simulink model "buck_pv"  (R2024a)
settings: Solver=FixedStepDiscrete  StartTime=0  StopTime=0.3  FixedStep=(1/150000)/100  RelTol=1e-3
model workspace (MAT data in the model file):
  Var = 20
values from neighbouring files (symbols this model uses):
  ki_0 = -mk*sin(thetak)*wcg_f    [Projeto_PI_Buck_PV_200W.m]    (also in Projeto_PI_Buck_PV_330W.m)
  kp_0 = mk*cos(thetak)    [Projeto_PI_Buck_PV_200W.m]    (also in Projeto_PI_Buck_PV_330W.m)
libraries: spsSeriesRLCBranchLib x6, spsDiodeLib x4, spsMeanLib x4, spsCurrentMeasurementLib x2, spsDCVoltageSourceLib x2, spsGroundLib x2, spsMosfetLib x2, spsPVArrayLib x2, spsPWMGeneratorDCDCLib x2, spsVoltageMeasurementLib x2, fuzblock x1, spspowerguiLib x1
settings Model: Creator=mario  LastModifiedBy=mario
settings SolverCC: MaxConsecutiveMinStep=10  ZeroCrossAlgorithm=Adaptive  SolverResetMethod=Robust
settings DebuggingCC: IgnoredZcDiagnostic=none
settings ModelReferenceCC: EnableRefExpFcnMdlSchedulingChecks=on
settings RTWCC: GPUComputeCapability=3.5

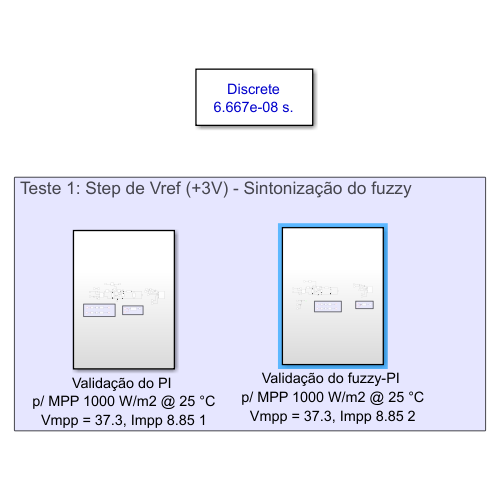
[thumbnail: Simulink's stored preview of the top-level diagram]
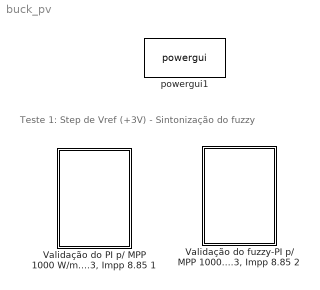
== system buck_pv ==
  note: Teste 1: Step de Vref (+3V) - Sintonização do fuzzy
  "Validação do PI p/ MPP 1000 W/m2 @ 25 °C Vmpp = 37.3, Impp 8.85 1" : Subsystem
  "Validação do fuzzy-PI p/ MPP 1000 W/m2 @ 25 °C Vmpp = 37.3, Impp 8.85 2" : Subsystem
  powergui1 : spspowerguiLib/powergui  Priority=1  SimulationMode=Discrete  SampleTime=(1/150000)/100  frequency=60  Iterations=50  frequencyindice=0  Pbase=100e6  ErrMax=1e-4  UnitsV=kV  UnitsW=MW  buscounter=0  FunctionMessages=off  echomessages=off  EnableUseOfTLC=off  CurrentSourceSwitches=off  DisableSnubberDevices=on  DisableRonSwitches=off  DisableVfSwitches=off  DisplayEquations=off  AutomaticDiscreteSolvers=off  SolverType=Tustin/Backward Euler (TBE)  Interpol=off  ExternalGateDelay=off  methode=off  Ts=100  x0status=blocks  SPID=on  SwTol=0  HookPort=off  NonlinearTolerance=1e-4  nMaxIteration=100  ContinueOnMaxIteration=on  RestoreLinks=warning  ResistiveCurrentMeasurement=off  Frange=[0:2:500]  Ylog=off  Xlog=on  ShowGrid=off  save=off  variable=ZData  structure=0  ZoomFFT=off  StartTime=0.0  cycles=1  DisplayStyle=1  fundamental=60  FreqAxis=off  MaxFrequency=1000  frequencyindicesteady=1  RmsSteady=1  display=off

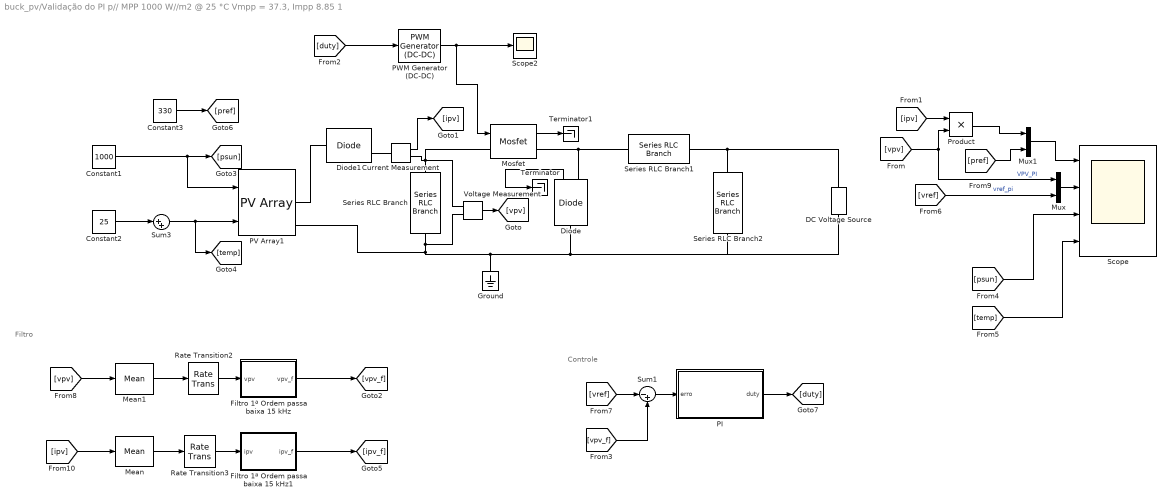
== system buck_pv/Validação do PI p// MPP 1000 W//m2 @ 25 °C Vmpp = 37.3, Impp 8.85 1 ==
  note: Controle
  note: Filtro
  Constant1 : Constant  Value=1000
  Constant2 : Constant  Value=25
  Constant3 : Constant  Value=330
  Current Measurement : spsCurrentMeasurementLib/Current Measurement  PhasorSimulation=off  OutputType=Complex  PSBequivalent=0
  DC Voltage Source : spsDCVoltageSourceLib/DC Voltage Source  Amplitude=12  Measurements=None
  Diode : spsDiodeLib/Diode  Ron=0.001  Lon=0  Vf=1  IC=0  UseSnubber=0  Rs=500  Cs=250e-9  Measurements=on
  Diode1 : spsDiodeLib/Diode  Ron=0.001  Lon=0  Vf=0.001  IC=0  UseSnubber=0  Rs=500  Cs=250e-9  Measurements=on
  Filtro 1ª Ordem passa baixa 15 kHz : MATLAB Function  TreatAsAtomicUnit=on
  Filtro 1ª Ordem passa baixa 15 kHz1 : MATLAB Function  TreatAsAtomicUnit=on
  Ground : spsGroundLib/Ground  LConnTagsString=a
  Mean : spsMeanLib/Mean  Freq=150e3  Vinit=0  Ts=(1/150000)/100
  Mean1 : spsMeanLib/Mean  Freq=150e3  Vinit=0  Ts=(1/150000)/100
  Mosfet : spsMosfetLib/Mosfet  Ron=6.5e-3  Lon=0  Rd=0.01  Vfd=0  IC=0  Rs=1e5  Cs=inf  Measurements=on
  Mux : Mux  Inputs=2
  Mux1 : Mux  Inputs=2
  PI : Subsystem
  PV Array1 : spsPVArrayLib/PV Array  Npar=1  Nser=1  PlotType=array @ 25 deg.C & specified irradiances  S_vec="[ 1000  800 600 400 200]"  Temp_C_vec=[ 50 40 30 20 10 ]  ModuleName=User-defined  PlotWhenSelected=off  Pm=330.105  Ncell=72  Voc=46.1  Isc=9.29  Vm=37.3  Im=8.85  beta_Voc_pc=-0.32  alpha_Isc_pc=0.05  beta_Voc=-0.14752  alpha_Isc=0.004645  IL=9.3231  I0=7.1464e-11  nI=0.97384  Rsh=1329.6875  Rs=0.38666  RobustModel=off  RobustCellTemperature=313.3991  BAL=on  Tc=1e-7  Tfilter=5e-5
  PWM Generator (DC-DC) : spsPWMGeneratorDCDCLib/PWM Generator (DC-DC)  Fsw=150000  Ts=1e-7
  Product : Product
  Rate Transition2 : RateTransition  OutPortSampleTime=1/150000
  Rate Transition3 : RateTransition  OutPortSampleTime=1/150000
  Scope : Scope  NumInputPorts=4
  Scope2 : Scope
  Series RLC Branch : spsSeriesRLCBranchLib/Series RLC Branch  LConnTagsString=__new0  RConnTagsString=__new0  BranchType=RC  Resistance=6.519e-3  Inductance=1e-3  SetiL0=off  InitialCurrent=0  Capacitance=2.7e-3  Setx0=off  InitialVoltage=37.3  Measurements=None
  Series RLC Branch1 : spsSeriesRLCBranchLib/Series RLC Branch  LConnTagsString=__new0  RConnTagsString=__new0  BranchType=RL  Resistance=3e-3  Inductance=22.109e-6  SetiL0=off  InitialCurrent=25.8056  Capacitance=1e-6  Setx0=off  InitialVoltage=0  Measurements=None
  Series RLC Branch2 : spsSeriesRLCBranchLib/Series RLC Branch  LConnTagsString=__new0  RConnTagsString=__new0  BranchType=RC  Resistance=35.2e-3  Inductance=1e-3  SetiL0=off  InitialCurrent=0  Capacitance=500e-6  Setx0=off  InitialVoltage=12  Measurements=None
  Sum1 : Sum  Inputs=|-+
  Sum3 : Sum  Inputs=|++
  Terminator : Terminator
  Terminator1 : Terminator
  Voltage Measurement : spsVoltageMeasurementLib/Voltage Measurement  PhasorSimulation=off  OutputType=Complex  PSBequivalent=0
  wires:
  Mux1/1 -> Scope/1
  [ipv] -> Product/1
  PWM Generator (DC-DC)/1 -> Scope2/1, Mosfet/1
  [vpv] -> Product/2, Mux/1  "VPV_PI"
  [duty] -> PWM Generator (DC-DC)/1
  Product/1 -> Mux1/1
  [pref] -> Mux1/2
  [psun] -> Scope/3
  [vref] -> Mux/2  "vref_pi"
  [temp] -> Scope/4
  Mux/1 -> Scope/2
  Diode/1 -> Terminator/1
  Mosfet/1 -> Terminator1/1
  Constant3/1 -> [pref]
  Voltage Measurement/1 -> [vpv]
  Current Measurement/1 -> [ipv]
  [vpv_f] -> Sum1/2
  [vref] -> Sum1/1
  Sum3/1 -> PV Array1/2, [temp]
  Constant2/1 -> Sum3/1
  Constant1/1 -> PV Array1/1, [psun]
  Sum1/1 -> PI/1(erro)
  PI/1(duty) -> [duty]
  Filtro 1ª Ordem passa baixa 15 kHz1/1(ipv_f) -> [ipv_f]
  Mean1/1 -> Rate Transition2/1
  Rate Transition2/1 -> Filtro 1ª Ordem passa baixa 15 kHz/1(vpv)
  Rate Transition3/1 -> Filtro 1ª Ordem passa baixa 15 kHz1/1(ipv)
  [vpv] -> Mean1/1
  Filtro 1ª Ordem passa baixa 15 kHz/1(vpv_f) -> [vpv_f]
  Mean/1 -> Rate Transition3/1
  [ipv] -> Mean/1
  connections:
  Series RLC Branch1/RConn1 -- DC Voltage Source/RConn1 -- Series RLC Branch2/LConn1
  Mosfet/LConn1 -- Current Measurement/RConn1 -- Voltage Measurement/LConn1 -- Series RLC Branch/LConn1
  DC Voltage Source/LConn1 -- Series RLC Branch2/RConn1 -- Diode/LConn1 -- Ground/LConn1 -- PV Array1/RConn2 -- Voltage Measurement/LConn2 -- Series RLC Branch/RConn1
  Mosfet/RConn1 -- Series RLC Branch1/LConn1 -- Diode/RConn1
  Diode1/RConn1 -- Current Measurement/LConn1
  PV Array1/RConn1 -- Diode1/LConn1

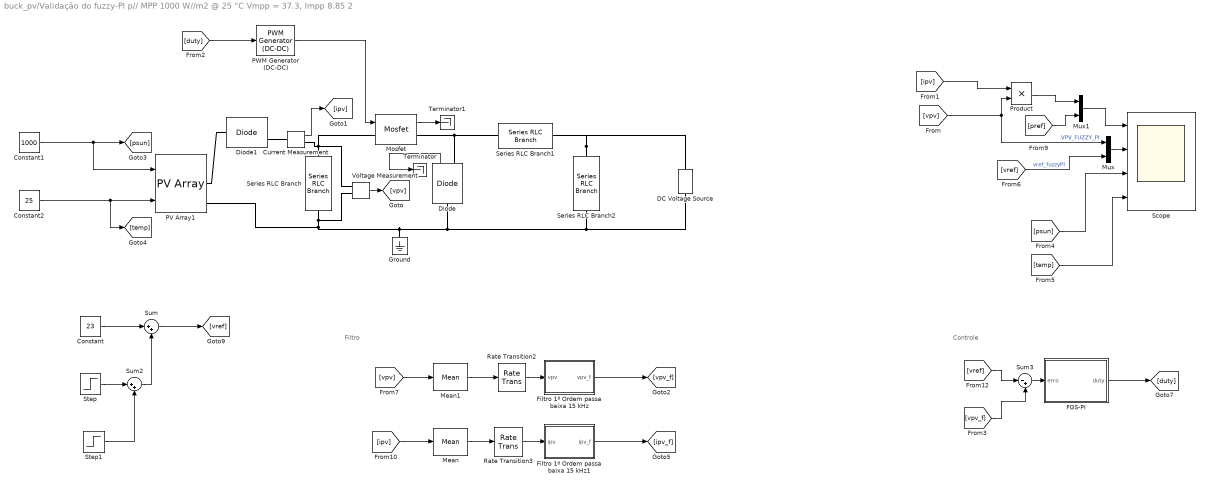
== system buck_pv/Validação do fuzzy-PI p// MPP 1000 W//m2 @ 25 °C Vmpp = 37.3, Impp 8.85 2 ==
  note: Controle
  note: Filtro
  Constant : Constant  Value=23
  Constant1 : Constant  Value=1000
  Constant2 : Constant  Value=25
  Current Measurement : spsCurrentMeasurementLib/Current Measurement  PhasorSimulation=off  OutputType=Complex  PSBequivalent=0
  DC Voltage Source : spsDCVoltageSourceLib/DC Voltage Source  Amplitude=12  Measurements=None
  Diode : spsDiodeLib/Diode  Ron=0.001  Lon=0  Vf=1  IC=0  UseSnubber=0  Rs=500  Cs=250e-9  Measurements=on
  Diode1 : spsDiodeLib/Diode  Ron=0.001  Lon=0  Vf=0.001  IC=0  UseSnubber=0  Rs=500  Cs=250e-9  Measurements=on
  "FGS-PI " : Subsystem
  Filtro 1ª Ordem passa baixa 15 kHz : MATLAB Function  TreatAsAtomicUnit=on
  Filtro 1ª Ordem passa baixa 15 kHz1 : MATLAB Function  TreatAsAtomicUnit=on
  Ground : spsGroundLib/Ground  LConnTagsString=a
  Mean : spsMeanLib/Mean  Freq=150e3  Vinit=0  Ts=(1/150000)/100
  Mean1 : spsMeanLib/Mean  Freq=150e3  Vinit=0  Ts=(1/150000)/100
  Mosfet : spsMosfetLib/Mosfet  Ron=0.15  Lon=0  Rd=0.01  Vfd=0  IC=0  Rs=1e5  Cs=inf  Measurements=on
  Mux : Mux  Inputs=2
  Mux1 : Mux  Inputs=2
  PV Array1 : spsPVArrayLib/PV Array  Npar=1  Nser=1  PlotType=array @ 1000 W/m2 & specified temperatures  S_vec="[ 1000  500  100 ]"  Temp_C_vec=[ 50 40 30 20 10 ]  ModuleName=User-defined  PlotWhenSelected=off  Pm=200.143  Ncell=45  Voc=32.9  Isc=8.21  Vm=26.3  Im=7.61  beta_Voc_pc=-0.123  alpha_Isc_pc=0.000318  beta_Voc=-0.040467  alpha_Isc=2.6108e-05  IL=8.2854  I0=9.6508e-16  nI=0.77673  Rsh=77.8782  Rs=0.47788  RobustModel=off  RobustCellTemperature=25  BAL=off  Tc=1e-7  Tfilter=(1/150000)*10
  PWM Generator (DC-DC) : spsPWMGeneratorDCDCLib/PWM Generator (DC-DC)  Fsw=150000  Ts=(1/150000)/100
  Product : Product
  Rate Transition2 : RateTransition  OutPortSampleTime=1/150000
  Rate Transition3 : RateTransition  OutPortSampleTime=1/150000
  Scope : Scope  NumInputPorts=4
  Series RLC Branch : spsSeriesRLCBranchLib/Series RLC Branch  LConnTagsString=__new0  RConnTagsString=__new0  BranchType=RC  Resistance=6.519e-3  Inductance=1e-3  SetiL0=off  InitialCurrent=0  Capacitance=2.7e-3  Setx0=on  InitialVoltage=37.3  Measurements=None
  Series RLC Branch1 : spsSeriesRLCBranchLib/Series RLC Branch  LConnTagsString=__new0  RConnTagsString=__new0  BranchType=RL  Resistance=3e-3  Inductance=22.109e-6  SetiL0=on  InitialCurrent=25.8056  Capacitance=1e-6  Setx0=off  InitialVoltage=0  Measurements=None
  Series RLC Branch2 : spsSeriesRLCBranchLib/Series RLC Branch  LConnTagsString=__new0  RConnTagsString=__new0  BranchType=RC  Resistance=35.2e-3  Inductance=1e-3  SetiL0=off  InitialCurrent=0  Capacitance=500e-6  Setx0=on  InitialVoltage=12  Measurements=None
  Step : Step  Time=0.12  After=3  SampleTime=0
  Step1 : Step  Time=0.22  After=-3  SampleTime=0
  Sum : Sum  Inputs=|++
  Sum2 : Sum  Inputs=|++
  Sum3 : Sum  Inputs=|-+
  Terminator : Terminator
  Terminator1 : Terminator
  Voltage Measurement : spsVoltageMeasurementLib/Voltage Measurement  PhasorSimulation=off  OutputType=Complex  PSBequivalent=0
  wires:
  Mux/1 -> Scope/2
  [temp] -> Scope/4
  [vref] -> Mux/2  "vref_fuzzyPI"
  [psun] -> Scope/3
  [pref] -> Mux1/2
  Product/1 -> Mux1/1
  [vpv] -> Mux/1, Product/2  "VPV_FUZZY_PI"
  [ipv] -> Product/1
  Mux1/1 -> Scope/1
  Voltage Measurement/1 -> [vpv]
  Current Measurement/1 -> [ipv]
  Mosfet/1 -> Terminator1/1
  Diode/1 -> Terminator/1
  [duty] -> PWM Generator (DC-DC)/1
  PWM Generator (DC-DC)/1 -> Mosfet/1
  Sum2/1 -> Sum/2
  Step/1 -> Sum2/1
  Step1/1 -> Sum2/2
  Constant/1 -> Sum/1
  [vpv_f] -> Sum3/2
  [vpv] -> Mean1/1
  Mean1/1 -> Rate Transition2/1
  [ipv] -> Mean/1
  Mean/1 -> Rate Transition3/1
  [vref] -> Sum3/1
  Sum/1 -> [vref]
  Constant2/1 -> PV Array1/2, [temp]
  Sum3/1 -> "FGS-PI "/1(erro)
  "FGS-PI "/1(duty) -> [duty]
  Filtro 1ª Ordem passa baixa 15 kHz/1(vpv_f) -> [vpv_f]
  Filtro 1ª Ordem passa baixa 15 kHz1/1(ipv_f) -> [ipv_f]
  Constant1/1 -> PV Array1/1, [psun]
  Rate Transition2/1 -> Filtro 1ª Ordem passa baixa 15 kHz/1(vpv)
  Rate Transition3/1 -> Filtro 1ª Ordem passa baixa 15 kHz1/1(ipv)
  connections:
  Series RLC Branch2/RConn1 -- Ground/LConn1 -- PV Array1/RConn2 -- Voltage Measurement/LConn2 -- Series RLC Branch/RConn1 -- Diode/LConn1 -- DC Voltage Source/LConn1
  Series RLC Branch/LConn1 -- Mosfet/LConn1 -- Current Measurement/RConn1 -- Voltage Measurement/LConn1
  Diode/RConn1 -- Mosfet/RConn1 -- Series RLC Branch1/LConn1
  Series RLC Branch2/LConn1 -- Series RLC Branch1/RConn1 -- DC Voltage Source/RConn1
  Diode1/RConn1 -- Current Measurement/LConn1
  Diode1/LConn1 -- PV Array1/RConn1

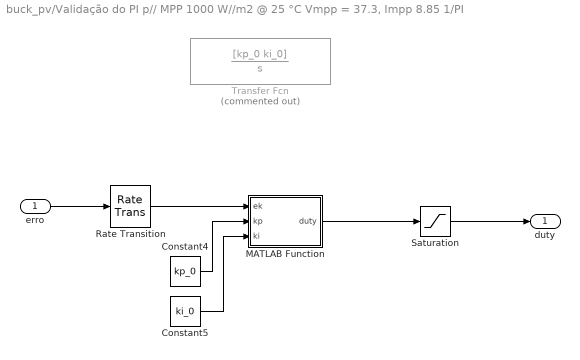
== system buck_pv/Validação do PI p// MPP 1000 W//m2 @ 25 °C Vmpp = 37.3, Impp 8.85 1/PI ==
  erro : Inport
  Constant4 : Constant  Value=kp_0
  Constant5 : Constant  Value=ki_0
  MATLAB Function : MATLAB Function  TreatAsAtomicUnit=on
  Rate Transition : RateTransition  OutPortSampleTime=1/100000
  Saturation : Saturate  UpperLimit=1  LowerLimit=0
  Transfer Fcn : TransferFcn  Commented=on  Numerator=[kp_0 ki_0]  Denominator=[1 0]
  duty : Outport
  wires:
  Saturation/1 -> duty/1
  Constant4/1 -> MATLAB Function/2(kp)
  Constant5/1 -> MATLAB Function/3(ki)
  MATLAB Function/1(duty) -> Saturation/1
  erro/1 -> Rate Transition/1
  Rate Transition/1 -> MATLAB Function/1(ek)

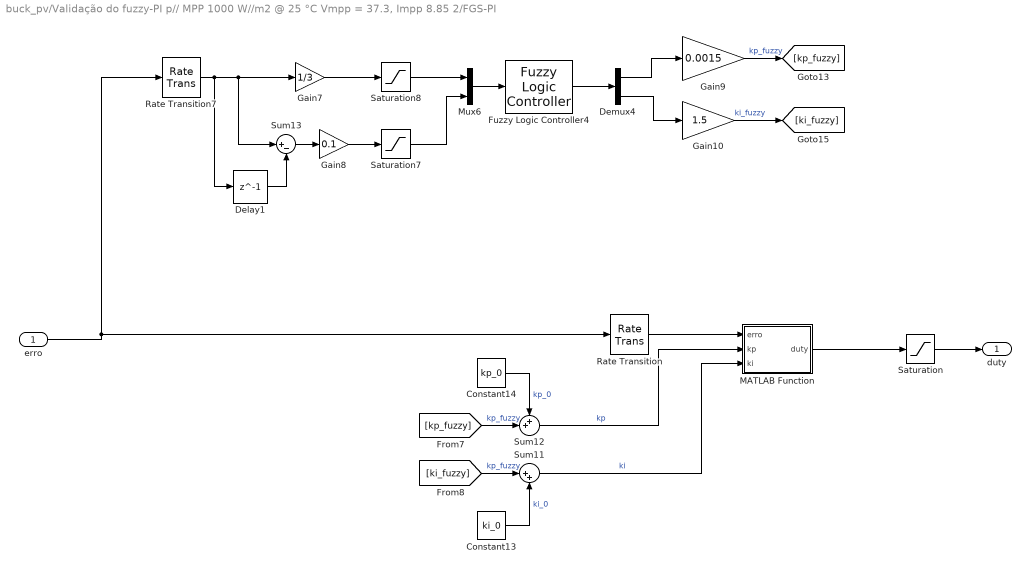
== system buck_pv/Validação do fuzzy-PI p// MPP 1000 W//m2 @ 25 °C Vmpp = 37.3, Impp 8.85 2/FGS-PI  ==
  erro : Inport
  Constant13 : Constant  Value=ki_0
  Constant14 : Constant  Value=kp_0
  Delay1 : Delay  DelayLength=1
  Demux4 : Demux  Outputs=2
  Fuzzy Logic Controller4 : fuzblock/Fuzzy Logic  Controller  FIS=FLS_FGS_PI  OutputSampleNumber=101  DataType=double  FuzzifiedInputs=off  RuleFiringStrengths=off  RuleOutputs=off  AggregatedOutputs=off  SimulateUsing=Interpreted execution  OutOfRangeInputValueMessage=warning  NoRuleFiredMessage=warning  EmptyOutputFuzzySetMessage=warning
  Gain10 : Gain  Gain=1.5
  Gain7 : Gain  Gain=1/3
  Gain8 : Gain  Gain=0.1
  Gain9 : Gain  Gain=0.0015
  MATLAB Function : MATLAB Function  TreatAsAtomicUnit=on
  Mux6 : Mux  Inputs=2
  Rate Transition : RateTransition  OutPortSampleTime=1/150000
  Rate Transition7 : RateTransition  OutPortSampleTime=20e-6
  Saturation : Saturate  UpperLimit=1  LowerLimit=0
  Saturation7 : Saturate  UpperLimit=1  LowerLimit=-1
  Saturation8 : Saturate  UpperLimit=1  LowerLimit=-1
  Sum11 : Sum  Inputs=|++
  Sum12 : Sum  Inputs=++|
  Sum13 : Sum  Inputs=|+-
  duty : Outport
  wires:
  [kp_fuzzy] -> Sum12/2  "kp_fuzzy"
  [ki_fuzzy] -> Sum11/1  "kp_fuzzy"
  Sum13/1 -> Gain8/1
  Gain7/1 -> Saturation8/1
  Gain9/1 -> [kp_fuzzy]  "kp_fuzzy"
  erro/1 -> Rate Transition/1, Rate Transition7/1
  Gain8/1 -> Saturation7/1
  Delay1/1 -> Sum13/2
  Constant13/1 -> Sum11/2  "ki_0"
  Constant14/1 -> Sum12/1  "kp_0"
  Fuzzy Logic Controller4/1 -> Demux4/1
  Saturation7/1 -> Mux6/2
  Demux4/1 -> Gain9/1
  Saturation8/1 -> Mux6/1
  Gain10/1 -> [ki_fuzzy]  "ki_fuzzy"
  Rate Transition7/1 -> Delay1/1, Sum13/1, Gain7/1
  Mux6/1 -> Fuzzy Logic Controller4/1
  Demux4/2 -> Gain10/1
  Rate Transition/1 -> MATLAB Function/1(erro)
  Sum12/1 -> MATLAB Function/2(kp)  "kp"
  Sum11/1 -> MATLAB Function/3(ki)  "ki"
  MATLAB Function/1(duty) -> Saturation/1
  Saturation/1 -> duty/1

== matlab function buck_pv/Validação do PI p// MPP 1000 W//m2 @ 25 °C Vmpp = 37.3, Impp 8.85 1/Filtro 1ª Ordem passa baixa 15 kHz1 ==
  data: ipv input; ipv_f output
function ipv_f = fcn(ipv)

%Valores p/ fc = 15 kHz
% b0 = 0.23905722;
% b1 = 0.23905722;
% a1 = -0.52188555;

%Valores p/ fc = 1.5 kHz
b0 = 0.030459028;
b1 = 0.030459028;
a1 = -0.93908194;

persistent ipv1 ipv_f1

if(isempty(ipv1)) ipv1=0; end
if(isempty(ipv_f1)) ipv_f1=0; end

ipv_f = (b0*ipv)+(b1*ipv1)-(a1*ipv_f1);
ipv1 = ipv;
ipv_f1 = ipv_f;

== matlab function buck_pv/Validação do PI p// MPP 1000 W//m2 @ 25 °C Vmpp = 37.3, Impp 8.85 1/PI/MATLAB Function ==
  settings: updateMethod=DISCRETE
  data: ek input; duty output; kp input; ki input
function duty = fcn(ek, kp, ki)

persistent uk_1 ek_1 Ik_1

if(isempty(uk_1)) uk_1=0; end
if(isempty(ek_1)) ek_1=0; end
if(isempty(Ik_1)) Ik_1=0; end

Ts = (1/100e3);
Ak = (ek + ek_1)/2*Ts;
Ik = Ik_1 + Ak;

u_PI = kp*ek + ki*Ik;

ek_1 = ek;
uk_1 = u_PI;
Ik_1 = Ik;

duty = u_PI;

== matlab function buck_pv/Validação do fuzzy-PI p// MPP 1000 W//m2 @ 25 °C Vmpp = 37.3, Impp 8.85 2/FGS-PI /MATLAB Function ==
  settings: updateMethod=DISCRETE
  data: erro input; duty output; kp input; ki input
function duty = fcn(erro, kp, ki)

persistent uk_1 ek_1 erro1 erro_f1
if(isempty(uk_1)) uk_1=0; end
if(isempty(ek_1)) ek_1=0; end


ek = erro;

Ts = (1/150e3);
A = kp+(ki*Ts/2);
B = kp - (ki*Ts/2);

u_PI = A*ek - B*ek_1 + uk_1;

ek_1 = ek;
uk_1 = u_PI;

duty = u_PI;

== matlab function buck_pv/Validação do fuzzy-PI p// MPP 1000 W//m2 @ 25 °C Vmpp = 37.3, Impp 8.85 2/Filtro 1ª Ordem passa baixa 15 kHz ==
  data: vpv input; vpv_f output
function vpv_f = fcn(vpv)

%Valores p/ fc = 15 kHz
% b0 = 0.23905722;
% b1 = 0.23905722;
% a1 = -0.52188555;

%Valores p/ fc = 1.5 kHz
b0 = 0.030459028;
b1 = 0.030459028;
a1 = -0.93908194;

persistent vpv1 vpv_f1

if(isempty(vpv1)) vpv1=0; end
if(isempty(vpv_f1)) vpv_f1=0; end

vpv_f = (b0*vpv)+(b1*vpv1)-(a1*vpv_f1);
vpv1 = vpv;
vpv_f1 = vpv_f;

== matlab function buck_pv/Validação do fuzzy-PI p// MPP 1000 W//m2 @ 25 °C Vmpp = 37.3, Impp 8.85 2/Filtro 1ª Ordem passa baixa 15 kHz1 ==
  data: ipv input; ipv_f output
function ipv_f = fcn(ipv)

%Valores p/ fc = 15 kHz
% b0 = 0.23905722;
% b1 = 0.23905722;
% a1 = -0.52188555;

%Valores p/ fc = 1.5 kHz
b0 = 0.030459028;
b1 = 0.030459028;
a1 = -0.93908194;

persistent ipv1 ipv_f1

if(isempty(ipv1)) ipv1=0; end
if(isempty(ipv_f1)) ipv_f1=0; end

ipv_f = (b0*ipv)+(b1*ipv1)-(a1*ipv_f1);
ipv1 = ipv;
ipv_f1 = ipv_f;

== matlab function buck_pv/Validação do PI p// MPP 1000 W//m2 @ 25 °C Vmpp = 37.3, Impp 8.85 1/Filtro 1ª Ordem passa baixa 15 kHz ==
  data: vpv input; vpv_f output
function vpv_f = fcn(vpv)

%Valores p/ fc = 15 kHz
% b0 = 0.23905722;
% b1 = 0.23905722;
% a1 = -0.52188555;

%Valores p/ fc = 1.5 kHz
b0 = 0.030459028;
b1 = 0.030459028;
a1 = -0.93908194;

persistent vpv1 vpv_f1

if(isempty(vpv1)) vpv1=0; end
if(isempty(vpv_f1)) vpv_f1=0; end

vpv_f = (b0*vpv)+(b1*vpv1)-(a1*vpv_f1);
vpv1 = vpv;
vpv_f1 = vpv_f;
